simulink model "Test"  (R2019b)
settings: Solver=FixedStepAuto  StartTime=0.0  StopTime=10.0  FixedStep=0.005  RelTol=1e-3
values from neighbouring files (symbols this model uses):
  unbroken = 0    [AplysiaFeeding.m]    (also in AplysiaFeeding_MATLAB.m = 1)
undefined symbols (not defined in the file or in its folder): force_on_object, grasper_friction_state, init_obj, jaw_friction_state, x_g, x_h
(part 1 of 2)
settings Model: Creator=mecha  LastModifiedBy=aslakshm

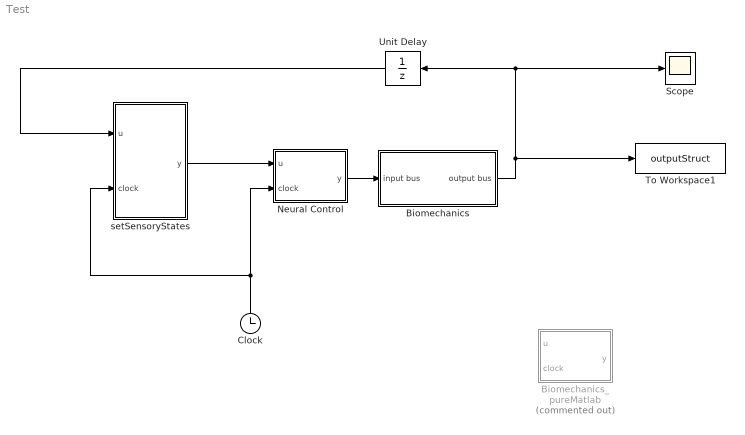
== system Test ==
  Biomechanics : Subsystem
  Biomechanics_pureMatlab : MATLAB Function  Commented=on  TreatAsAtomicUnit=on
  Clock : Clock
  Neural Control : MATLAB Function  TreatAsAtomicUnit=on
  Scope : Scope
  To Workspace1 : ToWorkspace  VariableName=outputStruct  SaveFormat=Timeseries  SampleTime=-1
  Unit Delay : UnitDelay  InitialCondition=init_obj  SampleTime=-1  HasFrameUpgradeWarning=on
  setSensoryStates : MATLAB Function  TreatAsAtomicUnit=on
  wires:
  Clock/1 -> Neural Control/2(clock), setSensoryStates/2(clock)
  Neural Control/1(y) -> Biomechanics/1(input bus)
  Biomechanics/1(output bus) -> To Workspace1/1, Unit Delay/1, Scope/1
  setSensoryStates/1(y) -> Neural Control/1(u)
  Unit Delay/1 -> setSensoryStates/1(u)

== system Test/Biomechanics ==
  input bus : Inport
  Bus Assignment : BusAssignment  AssignedSignals=x_g,x_h,force_on_object,unbroken,jaw_friction_state,grasper_friction_state
  Bus Selector1 : BusSelector  OutputSignals=x_g
  Bus Selector10 : BusSelector  OutputSignals=T_I2
  Bus Selector2 : BusSelector  OutputSignals=x_h
  Bus Selector3 : BusSelector  OutputSignals=fixation_type
  Bus Selector4 : BusSelector  OutputSignals=unbroken
  Bus Selector5 : BusSelector  OutputSignals=sens_mechanical_grasper
  Bus Selector6 : BusSelector  OutputSignals=P_I3_anterior
  Bus Selector7 : BusSelector  OutputSignals=P_I4
  Bus Selector8 : BusSelector  OutputSignals=T_hinge
  Bus Selector9 : BusSelector  OutputSignals=T_I3
  Subsystem : Subsystem
  output bus : Outport
  wires:
  Subsystem/3(Force_On_Object) -> Bus Assignment/4
  Bus Selector1/1 -> Subsystem/1(x_g)  "<x_g>"
  input bus/1 -> Bus Selector10/1, Bus Selector9/1, Bus Selector8/1, Bus Selector7/1, Bus Selector6/1, Bus Selector5/1, Bus Selector4/1, Bus Selector3/1, Bus Selector2/1, Bus Selector1/1, Bus Assignment/1
  Bus Selector2/1 -> Subsystem/2(x_h)  "<x_h>"
  Bus Selector5/1 -> Subsystem/5(sens_mechanical_grasper)  "<sens_mechanical_grasper>"
  Bus Assignment/1 -> output bus/1
  Bus Selector6/1 -> Subsystem/6(P_I3_anterior)  "<P_I3_anterior>"
  Bus Selector7/1 -> Subsystem/7(P_I4)  "<P_I4>"
  Subsystem/2(x_h_out) -> Bus Assignment/3
  Bus Selector3/1 -> Subsystem/3(fixation_type)  "<fixation_type>"
  Subsystem/1(x_g_out) -> Bus Assignment/2
  Bus Selector10/1 -> Subsystem/10(T_I2)  "<T_I2>"
  Bus Selector8/1 -> Subsystem/8(T_hinge)  "<T_hinge>"
  Bus Selector4/1 -> Subsystem/4(unbroken)  "<unbroken>"
  Bus Selector9/1 -> Subsystem/9(T_I3)  "<T_I3>"
  Subsystem/4(unbroken_out) -> Bus Assignment/5
  Subsystem/5(jaw friction state) -> Bus Assignment/6
  Subsystem/6(grasper_friction_state) -> Bus Assignment/7

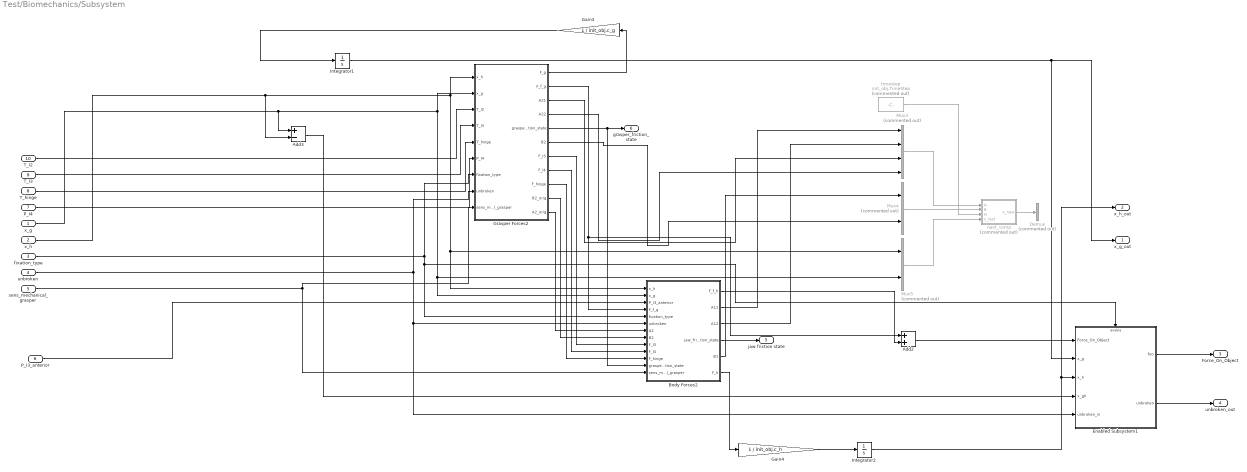
== system Test/Biomechanics/Subsystem ==
  x_g : Inport
  x_h : Inport  Port=2
  fixation_type : Inport  Port=3
  unbroken : Inport  Port=4
  sens_mechanical_grasper : Inport  Port=5
  P_I3_anterior : Inport  Port=6
  P_I4 : Inport  Port=7
  T_hinge : Inport  Port=8
  T_I3 : Inport  Port=9
  T_I2 : Inport  Port=10
  Add2 : Sum
  Add3 : Sum  Inputs=+-
  Body Forces2 : Subsystem
  Demux : Demux  Commented=on  Outputs=2
  Enabled Subsystem1 : Subsystem  TreatAsAtomicUnit=on
  Gain3 : Gain  Gain=1 / init_obj.c_g
  Gain4 : Gain  Gain=1 / init_obj.c_h
  Grasper Forces2 : Subsystem
  Integrator1 : Integrator  InitialCondition=init_obj.x_g_init
  Integrator2 : Integrator  InitialCondition=init_obj.x_h_init
  Mux3 : Mux  Commented=on
  Mux4 : Mux  Commented=on  Inputs=2
  Mux5 : Mux  Commented=on  Inputs=2
  next_comp : MATLAB Function  Commented=on  TreatAsAtomicUnit=on
  timestep : Constant  Commented=on  Value=init_obj.TimeStep
  x_g_out : Outport
  x_h_out : Outport  Port=2
  Force_On_Object : Outport  Port=3
  unbroken_out : Outport  Port=4
  jaw friction state : Outport  Port=5
  grasper_friction_state : Outport  Port=6
  wires:
  P_I4/1 -> Grasper Forces2/6(P_I4)
  Add2/1 -> Enabled Subsystem1/1(Force_On_Object)
  Body Forces2/3(A12) -> Mux3/2
  next_comp/1(x_new) -> Demux/1
  timestep/1 -> next_comp/3(ts)
  Add3/1 -> Enabled Subsystem1/4(x_gh)
  Body Forces2/2(A11) -> Mux3/1
  P_I3_anterior/1 -> Body Forces2/3(P_I3_anterior)
  Mux3/1 -> next_comp/1(A)
  Body Forces2/5(B1) -> Mux4/1
  T_I3/1 -> Grasper Forces2/4(T_I3)
  Grasper Forces2/8(F_I4) -> Body Forces2/10(F_I4)
  unbroken/1 -> Grasper Forces2/8(unbroken), Body Forces2/6(unbroken), Enabled Subsystem1/5(unbroken_in)
  T_hinge/1 -> Grasper Forces2/5(T_hinge)
  fixation_type/1 -> Grasper Forces2/7(fixation_type), Body Forces2/5(fixation_type), Enabled Subsystem1/Enable
  Grasper Forces2/2(F_f_g) -> Body Forces2/4(F_f_g), Add2/1
  Grasper Forces2/7(F_I3) -> Body Forces2/9(F_I3)
  Body Forces2/1(F_f_h) -> Add2/2
  T_I2/1 -> Grasper Forces2/3(T_I2)
  x_g/1 -> Add3/1, Grasper Forces2/2(x_g), Body Forces2/2(x_g), Mux5/2
  Grasper Forces2/10(B2_orig) -> Body Forces2/8(B2)
  sens_mechanical_grasper/1 -> Body Forces2/13(sens_mechanical_grasper), Grasper Forces2/9(sens_mechanical_grasper)
  Grasper Forces2/5(grasper_friction_state) -> Body Forces2/12(grasper_friction_state), grasper_friction_state/1
  Mux4/1 -> next_comp/2(B)
  Grasper Forces2/4(A22) -> Mux3/4
  Grasper Forces2/6(B2) -> Mux4/2
  x_h/1 -> Add3/2, Grasper Forces2/1(x_h), Body Forces2/1(x_h), Mux5/1
  Enabled Subsystem1/1(foo) -> Force_On_Object/1
  Grasper Forces2/3(A21) -> Mux3/3
  Grasper Forces2/11(A2_orig) -> Body Forces2/7(A2)
  Mux5/1 -> next_comp/4(x_last)
  Enabled Subsystem1/2(unbroken) -> unbroken_out/1
  Body Forces2/4(jaw_friction_state) -> jaw friction state/1
  Grasper Forces2/9(F_hinge) -> Body Forces2/11(F_hinge)
  Gain3/1 -> Integrator1/1
  Grasper Forces2/1(F_g) -> Gain3/1
  Integrator1/1 -> Enabled Subsystem1/2(x_g), x_g_out/1
  Body Forces2/6(F_h) -> Gain4/1
  Gain4/1 -> Integrator2/1
  Integrator2/1 -> Enabled Subsystem1/3("x_h "), x_h_out/1

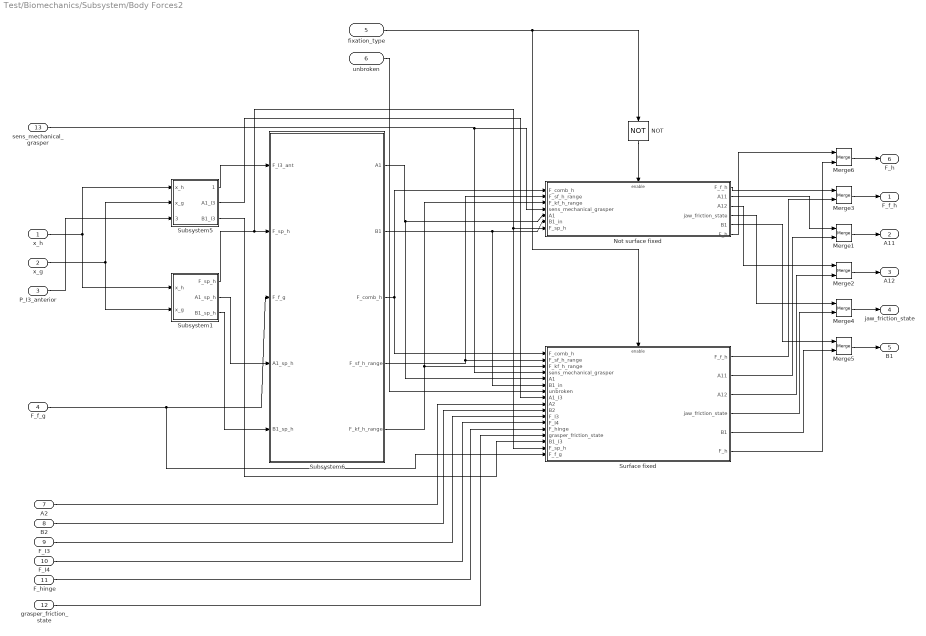
== system Test/Biomechanics/Subsystem/Body Forces2 ==
  x_h : Inport
  x_g : Inport  Port=2
  P_I3_anterior : Inport  Port=3
  F_f_g : Inport  Port=4
  fixation_type : Inport  Port=5
  unbroken : Inport  Port=6
  A2 : Inport  Port=7
  B2 : Inport  Port=8
  F_I3 : Inport  Port=9
  F_I4 : Inport  Port=10
  F_hinge : Inport  Port=11
  grasper_friction_state : Inport  Port=12
  sens_mechanical_grasper : Inport  Port=13
  Merge{1..6} (6 alike) : Merge
  NOT : Logic  Operator=NOT  IconShape=distinctive  AllPortsSameDT=off  OutDataTypeStr=boolean
  Not surface fixed : Subsystem
  Subsystem1 : Subsystem
  Subsystem5 : Subsystem
  Subsystem6 : Subsystem
  Surface fixed : Subsystem
  F_f_h : Outport
  A11 : Outport  Port=2
  A12 : Outport  Port=3
  jaw_friction_state : Outport  Port=4
  B1 : Outport  Port=5
  F_h : Outport  Port=6
  wires:
  Subsystem5/1(F_I3_ant) -> Subsystem6/1(F_I3_ant)
  Subsystem1/1(F_sp_h) -> Surface fixed/16(F_sp_h), Not surface fixed/7(F_sp_h), Subsystem6/2(F_sp_h)
  x_g/1 -> Subsystem1/2(x_g), Subsystem5/2(x_g)
  x_h/1 -> Subsystem1/1(x_h), Subsystem5/1(x_h)
  F_f_g/1 -> Surface fixed/17(F_f_g), Subsystem6/3(F_f_g)
  Subsystem6/4(F_sf_h_range) -> Not surface fixed/2(F_sf_h_range), Surface fixed/2(F_sf_h_range)
  Subsystem6/5(F_kf_h_range) -> Not surface fixed/3(F_kf_h_range), Surface fixed/3(F_kf_h_range)
  Subsystem6/1(A1) -> Surface fixed/5(A1), Not surface fixed/5(A1)
  Subsystem6/3(F_comb_h) -> Surface fixed/1(F_comb_h), Not surface fixed/1(F_comb_h)
  NOT/1 -> Not surface fixed/Enable
  fixation_type/1 -> Surface fixed/Enable, NOT/1
  Merge4/1 -> jaw_friction_state/1
  Merge1/1 -> A11/1
  Merge2/1 -> A12/1
  Merge5/1 -> B1/1
  Merge3/1 -> F_f_h/1
  Surface fixed/5(B1) -> Merge5/2
  Not surface fixed/5(B1) -> Merge5/1
  Surface fixed/4(jaw_friction_state) -> Merge4/2
  Not surface fixed/4(jaw_friction_state) -> Merge4/1
  Surface fixed/3(A12) -> Merge2/2
  Not surface fixed/3(A12) -> Merge2/1
  Surface fixed/2(A11) -> Merge1/2
  Not surface fixed/2(A11) -> Merge1/1
  Surface fixed/1(F_f_h) -> Merge3/2
  Not surface fixed/1(F_f_h) -> Merge3/1
  unbroken/1 -> Surface fixed/7(unbroken)
  Subsystem5/2(A1_I3) -> Surface fixed/8(A1_I3)
  Subsystem5/3(B1_I3) -> Surface fixed/15(B1_I3)
  Subsystem1/2(A1_sp_h) -> Subsystem6/4(A1_sp_h)
  Subsystem1/3(B1_sp_h) -> Subsystem6/5(B1_sp_h)
  A2/1 -> Surface fixed/9(A2)
  B2/1 -> Surface fixed/10(B2)
  grasper_friction_state/1 -> Surface fixed/14(grasper_friction_state)
  Subsystem6/2(B1) -> Surface fixed/6(B1_in), Not surface fixed/6(B1_in)
  P_I3_anterior/1 -> Subsystem5/3(P_I3_anterior)
  F_hinge/1 -> Surface fixed/13(F_hinge)
  F_I3/1 -> Surface fixed/11(F_I3)
  F_I4/1 -> Surface fixed/12(F_I4)
  sens_mechanical_grasper/1 -> Surface fixed/4(sens_mechanical_grasper), Not surface fixed/4(sens_mechanical_grasper)
  Merge6/1 -> F_h/1
  Not surface fixed/6(F_h) -> Merge6/1
  Surface fixed/6(F_h) -> Merge6/2

== system Test/Biomechanics/Subsystem/Enabled Subsystem1 ==
  Force_On_Object : Inport
  x_g : Inport  Port=2
  "x_h " : Inport  Port=3
  x_gh : Inport  Port=4
  unbroken_in : Inport  Port=5
  Enable : EnablePort
  AND : Logic  Inputs=3  IconShape=distinctive  AllPortsSameDT=off  OutDataTypeStr=boolean
  Add : Sum  Inputs=+-
  Constant : Constant  Value=init_obj.seaweed_strength
  Constant1 : Constant  Value=0.3
  Enabled Subsystem : Subsystem  TreatAsAtomicUnit=on
  Enabled Subsystem1 : Subsystem  TreatAsAtomicUnit=on
  GreaterThan : RelationalOperator  Operator=>  OutDataTypeStr=boolean  RndMeth=Simplest
  Less Than : RelationalOperator  Operator=<  OutDataTypeStr=boolean  RndMeth=Simplest
  Less Than1 : RelationalOperator  Operator=>  OutDataTypeStr=boolean  RndMeth=Simplest
  Merge : Merge
  NOT : Logic  Operator=NOT  IconShape=distinctive  AllPortsSameDT=off  OutDataTypeStr=boolean
  NOT1 : Logic  Operator=NOT  IconShape=distinctive  AllPortsSameDT=off  OutDataTypeStr=boolean
  Product : Product
  foo : Outport
  unbroken : Outport  Port=2
  wires:
  Force_On_Object/1 -> Product/1, GreaterThan/1
  Constant/1 -> GreaterThan/2
  x_g/1 -> Add/1
  "x_h "/1 -> Add/2
  x_gh/1 -> Less Than1/2, Less Than/1
  Constant1/1 -> Less Than/2
  Add/1 -> Less Than1/1
  unbroken_in/1 -> Enabled Subsystem1/2(unbroken_in), NOT/1
  Less Than1/1 -> AND/1
  Less Than/1 -> AND/2
  NOT/1 -> AND/3
  AND/1 -> Enabled Subsystem/Enable, NOT1/1
  NOT1/1 -> Enabled Subsystem1/Enable
  GreaterThan/1 -> Enabled Subsystem1/1(force_check)
  Merge/1 -> Product/2, unbroken/1
  Enabled Subsystem1/1(Out1) -> Merge/2
  Enabled Subsystem/1(Out1) -> Merge/1
  Product/1 -> foo/1

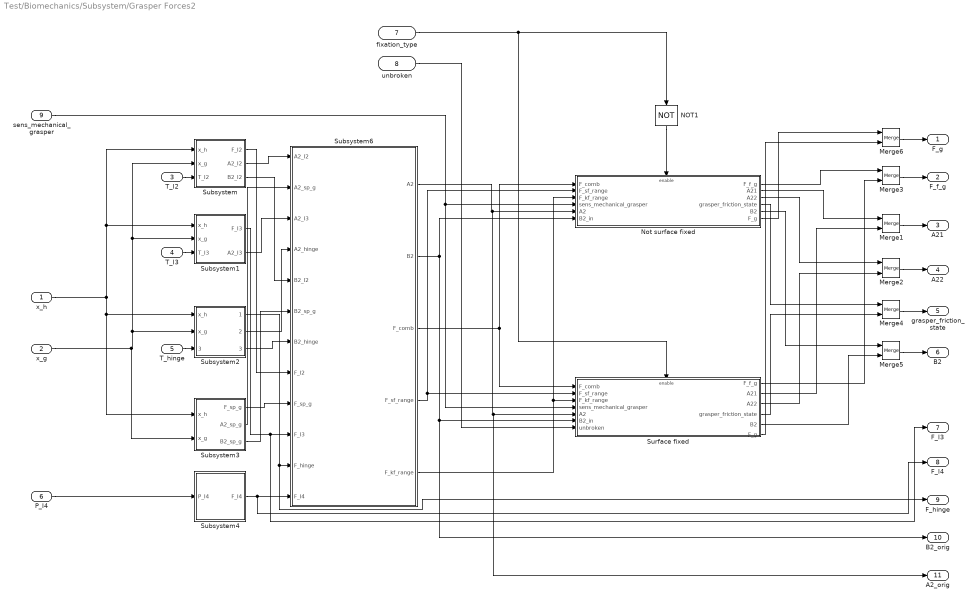
== system Test/Biomechanics/Subsystem/Grasper Forces2 ==
  x_h : Inport
  x_g : Inport  Port=2
  T_I2 : Inport  Port=3
  T_I3 : Inport  Port=4
  T_hinge : Inport  Port=5
  P_I4 : Inport  Port=6
  fixation_type : Inport  Port=7
  unbroken : Inport  Port=8
  sens_mechanical_grasper : Inport  Port=9
  Merge{1..6} (6 alike) : Merge
  NOT1 : Logic  Operator=NOT  IconShape=distinctive  AllPortsSameDT=off  OutDataTypeStr=boolean
  Not surface fixed : Subsystem
  Subsystem : Subsystem
  Subsystem1 : Subsystem
  Subsystem2 : Subsystem
  Subsystem3 : Subsystem
  Subsystem4 : Subsystem
  Subsystem6 : Subsystem
  Surface fixed : Subsystem
  F_g : Outport
  F_f_g : Outport  Port=2
  A21 : Outport  Port=3
  A22 : Outport  Port=4
  grasper_friction_state : Outport  Port=5
  B2 : Outport  Port=6
  F_I3 : Outport  Port=7
  F_I4 : Outport  Port=8
  F_hinge : Outport  Port=9
  B2_orig : Outport  Port=10
  A2_orig : Outport  Port=11
  wires:
  T_hinge/1 -> Subsystem2/3(T_hinge)
  x_h/1 -> Subsystem3/1(x_h), Subsystem2/1(x_h), Subsystem1/1(x_h), Subsystem/1(x_h)
  P_I4/1 -> Subsystem4/1(P_I4)
  x_g/1 -> Subsystem3/2(x_g), Subsystem1/2(x_g), Subsystem/2(x_g), Subsystem2/2(x_g)
  T_I3/1 -> Subsystem1/3(T_I3)
  T_I2/1 -> Subsystem/3(T_I2)
  Subsystem4/1(F_I4) -> F_I4/1, Subsystem6/12(F_I4)
  Subsystem/2(A2_I2) -> Subsystem6/1(A2_I2)
  Subsystem/1(F_I2) -> Subsystem6/8(F_I2)
  Subsystem/3(B2_I2) -> Subsystem6/5(B2_I2)
  Subsystem1/1(F_I3) -> F_I3/1, Subsystem6/10(F_I3)
  Subsystem3/1(F_sp_g) -> Subsystem6/9(F_sp_g)
  Subsystem3/2(A2_sp_g) -> Subsystem6/2(A2_sp_g)
  Subsystem3/3(B2_sp_g) -> Subsystem6/6(B2_sp_g)
  Subsystem2/1(F_hinge) -> F_hinge/1, Subsystem6/11(F_hinge)
  Subsystem2/3(B2_hinge) -> Subsystem6/7(B2_hinge)
  Subsystem2/2(A2_hinge) -> Subsystem6/4(A2_hinge)
  Subsystem1/2(A2_I3) -> Subsystem6/3(A2_I3)
  fixation_type/1 -> Surface fixed/Enable, NOT1/1
  unbroken/1 -> Surface fixed/7(unbroken)
  Subsystem6/1(A2) -> A2_orig/1, Surface fixed/5(A2), Not surface fixed/5(A2)
  Subsystem6/4(F_sf_range) -> Surface fixed/2(F_sf_range), Not surface fixed/2(F_sf_range)
  Subsystem6/5(F_kf_range) -> Not surface fixed/3(F_kf_range), Surface fixed/3(F_kf_range)
  sens_mechanical_grasper/1 -> Surface fixed/4(sens_mechanical_grasper), Not surface fixed/4(sens_mechanical_grasper)
  Merge1/1 -> A21/1
  Merge2/1 -> A22/1
  Merge4/1 -> grasper_friction_state/1
  Not surface fixed/1(F_f_g) -> Merge3/1
  Surface fixed/1(F_f_g) -> Merge3/2
  Not surface fixed/2(A21) -> Merge1/1
  Surface fixed/2(A21) -> Merge1/2
  Not surface fixed/3(A22) -> Merge2/1
  Surface fixed/3(A22) -> Merge2/2
  Not surface fixed/4(grasper_friction_state) -> Merge4/1
  Surface fixed/4(grasper_friction_state) -> Merge4/2
  Not surface fixed/5(B2) -> Merge5/1
  NOT1/1 -> Not surface fixed/Enable
  Subsystem6/2(B2) -> B2_orig/1, Surface fixed/6(B2_in), Not surface fixed/6(B2_in)
  Surface fixed/5(B2) -> Merge5/2
  Merge5/1 -> B2/1
  Subsystem6/3(F_comb) -> Surface fixed/1(F_comb), Not surface fixed/1(F_comb)
  Merge3/1 -> F_f_g/1
  Merge6/1 -> F_g/1
  Surface fixed/6(F_g) -> Merge6/2
  Not surface fixed/6(F_g) -> Merge6/1

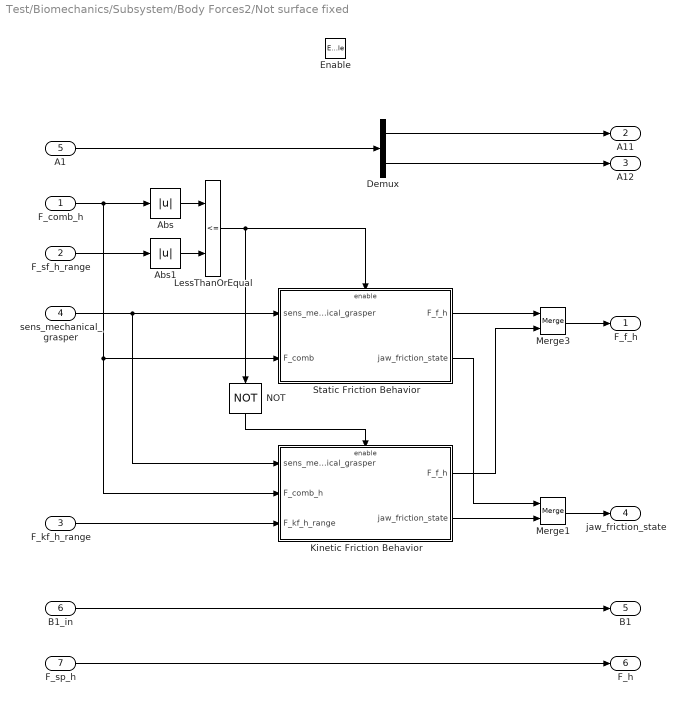
== system Test/Biomechanics/Subsystem/Body Forces2/Not surface fixed ==
  F_comb_h : Inport
  F_sf_h_range : Inport  Port=2
  F_kf_h_range : Inport  Port=3
  sens_mechanical_grasper : Inport  Port=4
  A1 : Inport  Port=5
  B1_in : Inport  Port=6
  F_sp_h : Inport  Port=7
  Enable : EnablePort
  Abs : Abs
  Abs1 : Abs
  Demux : Demux  Outputs=2
  Kinetic Friction Behavior : Subsystem
  LessThanOrEqual : RelationalOperator  Operator=<=  OutDataTypeStr=boolean  RndMeth=Simplest
  Merge1 : Merge
  Merge3 : Merge
  NOT : Logic  Operator=NOT  IconShape=distinctive  AllPortsSameDT=off  OutDataTypeStr=boolean
  Static Friction Behavior : Subsystem
  F_f_h : Outport
  A11 : Outport  Port=2
  A12 : Outport  Port=3
  jaw_friction_state : Outport  Port=4
  B1 : Outport  Port=5
  F_h : Outport  Port=6
  wires:
  A1/1 -> Demux/1
  Demux/2 -> A12/1
  Demux/1 -> A11/1
  F_comb_h/1 -> Kinetic Friction Behavior/2(F_comb_h), Static Friction Behavior/2(F_comb), Abs/1
  F_kf_h_range/1 -> Kinetic Friction Behavior/3(F_kf_h_range)
  F_sf_h_range/1 -> Abs1/1
  Abs/1 -> LessThanOrEqual/1
  Abs1/1 -> LessThanOrEqual/2
  LessThanOrEqual/1 -> NOT/1, Static Friction Behavior/Enable
  NOT/1 -> Kinetic Friction Behavior/Enable
  sens_mechanical_grasper/1 -> Kinetic Friction Behavior/1(sens_mechanical_grasper), Static Friction Behavior/1(sens_mechanical_grasper)
  Static Friction Behavior/1(F_f_h) -> Merge3/1
  Kinetic Friction Behavior/1(F_f_h) -> Merge3/2
  Kinetic Friction Behavior/2(jaw_friction_state) -> Merge1/2
  Static Friction Behavior/2(jaw_friction_state) -> Merge1/1
  Merge3/1 -> F_f_h/1
  Merge1/1 -> jaw_friction_state/1
  B1_in/1 -> B1/1
  F_sp_h/1 -> F_h/1

== system Test/Biomechanics/Subsystem/Body Forces2/Subsystem1 ==
  x_h : Inport
  x_g : Inport  Port=2
  Add2 : Sum
  Constant1 : Constant  Value=init_obj.x_h_ref
  Constant2 : Constant  Value=[-1 0]
  Constant3 : Constant  Value=init_obj.K_sp_h
  Dot Product1 : DotProduct  InputSameDT=on  OutDataTypeStr=Inherit: Inherit via internal rule
  Mux : Mux  Inputs=2
  Product1 : Product
  Product2 : Product
  Product3 : Product
  F_sp_h : Outport
  A1_sp_h : Outport  Port=2
  B1_sp_h : Outport  Port=3
  wires:
  Constant2/1 -> Product1/1, Dot Product1/1
  Dot Product1/1 -> Add2/2
  Mux/1 -> Dot Product1/2
  x_g/1 -> Mux/2
  x_h/1 -> Mux/1
  Product2/1 -> F_sp_h/1
  Add2/1 -> Product2/2
  Constant3/1 -> Product1/2, Product3/2, Product2/1
  Constant1/1 -> Product3/1, Add2/1
  Product1/1 -> A1_sp_h/1
  Product3/1 -> B1_sp_h/1

== system Test/Biomechanics/Subsystem/Body Forces2/Subsystem5 ==
  x_h : Inport
  x_g : Inport  Port=2
  P_I3_anterior : Inport  Port=3
  Add2 : Sum
  Constant1 : Constant
  Constant2 : Constant  Value=[1 -1]
  Constant3 : Constant  Value=init_obj.max_I3ant
  Dot Product : DotProduct  InputSameDT=on  OutDataTypeStr=Inherit: Inherit via internal rule
  Mux : Mux  Inputs=2
  Product1 : Product  Inputs=3
  Product2 : Product  Inputs=3
  Product3 : Product  Inputs=3
  F_I3_ant : Outport
  A1_I3 : Outport  Port=2
  B1_I3 : Outport  Port=3
  wires:
  Dot Product/1 -> Add2/2
  Mux/1 -> Dot Product/2
  x_g/1 -> Mux/2
  x_h/1 -> Mux/1
  Product2/1 -> F_I3_ant/1
  Add2/1 -> Product2/2
  Constant2/1 -> Product1/2, Dot Product/1
  Product1/1 -> A1_I3/1
  P_I3_anterior/1 -> Product3/3, Product1/3, Product2/3
  Constant1/1 -> Product3/2, Add2/1
  Constant3/1 -> Product3/1, Product1/1, Product2/1
  Product3/1 -> B1_I3/1

== system Test/Biomechanics/Subsystem/Body Forces2/Subsystem6 ==
  F_I3_ant : Inport
  F_sp_h : Inport  Port=2
  F_f_g : Inport  Port=3
  A1_sp_h : Inport  Port=4
  B1_sp_h : Inport  Port=5
  Add : Sum
  Gain1 : Gain  Gain=1 / init_obj.c_h
  Gain2 : Gain  Gain=init_obj.mu_s_h
  Gain3 : Gain  Gain=init_obj.mu_k_h
  Gain4 : Gain  Gain=1 / init_obj.c_h
  A1 : Outport
  B1 : Outport  Port=2
  F_comb_h : Outport  Port=3
  F_sf_h_range : Outport  Port=4
  F_kf_h_range : Outport  Port=5
  wires:
  Add/1 -> F_comb_h/1
  F_I3_ant/1 -> Gain2/1, Gain3/1
  Gain2/1 -> F_sf_h_range/1
  Gain3/1 -> F_kf_h_range/1
  F_sp_h/1 -> Add/1
  F_f_g/1 -> Add/2
  Gain4/1 -> A1/1
  A1_sp_h/1 -> Gain4/1
  Gain1/1 -> B1/1
  B1_sp_h/1 -> Gain1/1

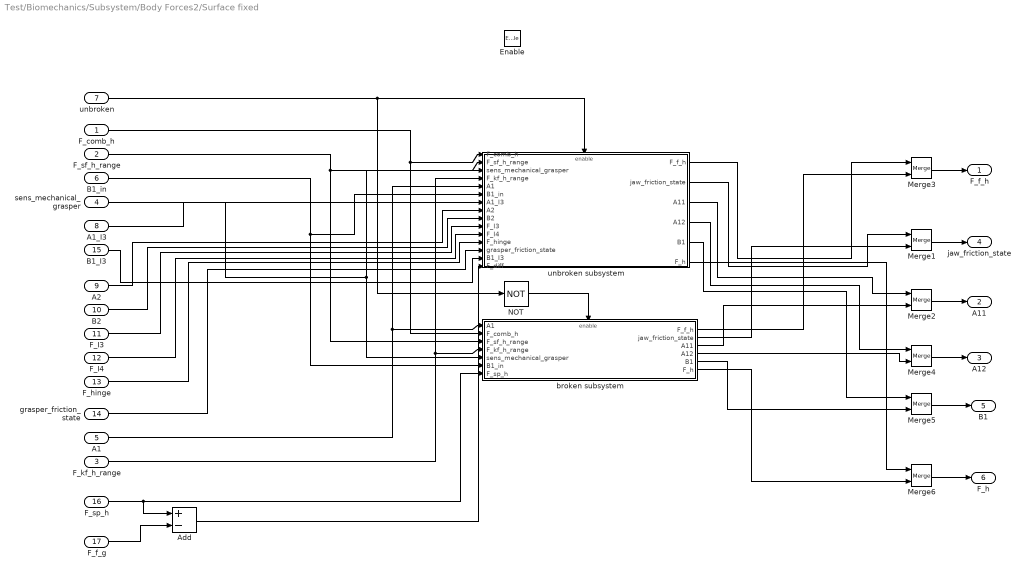
== system Test/Biomechanics/Subsystem/Body Forces2/Surface fixed ==
  F_comb_h : Inport
  F_sf_h_range : Inport  Port=2
  F_kf_h_range : Inport  Port=3
  sens_mechanical_grasper : Inport  Port=4
  A1 : Inport  Port=5
  B1_in : Inport  Port=6
  unbroken : Inport  Port=7
  A1_I3 : Inport  Port=8
  A2 : Inport  Port=9
  B2 : Inport  Port=10
  F_I3 : Inport  Port=11
  F_I4 : Inport  Port=12
  F_hinge : Inport  Port=13
  grasper_friction_state : Inport  Port=14
  B1_I3 : Inport  Port=15
  F_sp_h : Inport  Port=16
  F_f_g : Inport  Port=17
  Enable : EnablePort
  Add : Sum  Inputs=+-
  Merge{1..6} (6 alike) : Merge
  NOT : Logic  Operator=NOT  IconShape=distinctive  AllPortsSameDT=off  OutDataTypeStr=boolean
  broken subsystem : Subsystem
  unbroken subsystem : Subsystem
  F_f_h : Outport
  A11 : Outport  Port=2
  A12 : Outport  Port=3
  jaw_friction_state : Outport  Port=4
  B1 : Outport  Port=5
  F_h : Outport  Port=6
  wires:
  unbroken/1 -> NOT/1, unbroken subsystem/Enable
  NOT/1 -> broken subsystem/Enable
  F_comb_h/1 -> broken subsystem/2(F_comb_h), unbroken subsystem/1(F_comb_h)
  F_sf_h_range/1 -> broken subsystem/3(F_sf_h_range), unbroken subsystem/2(F_sf_h_range)
  A1/1 -> unbroken subsystem/5(A1), broken subsystem/1(A1)
  B1_in/1 -> broken subsystem/6(B1_in), unbroken subsystem/6(B1_in)
  Merge3/1 -> F_f_h/1
  Merge1/1 -> jaw_friction_state/1
  broken subsystem/1(F_f_h) -> Merge3/2
  unbroken subsystem/2(jaw_friction_state) -> Merge1/1
  broken subsystem/2(jaw_friction_state) -> Merge1/2
  Merge2/1 -> A11/1
  Merge4/1 -> A12/1
  unbroken subsystem/3(A11) -> Merge2/1
  broken subsystem/3(A11) -> Merge2/2
  unbroken subsystem/4(A12) -> Merge4/1
  broken subsystem/4(A12) -> Merge4/2
  unbroken subsystem/5(B1) -> Merge5/1
  F_kf_h_range/1 -> unbroken subsystem/4(F_kf_h_range), broken subsystem/4(F_kf_h_range)
  sens_mechanical_grasper/1 -> unbroken subsystem/3(sens_mechanical_grasper), broken subsystem/5(sens_mechanical_grasper)
  Merge5/1 -> B1/1
  broken subsystem/5(B1) -> Merge5/2
  unbroken subsystem/1(F_f_h) -> Merge3/1
  A1_I3/1 -> unbroken subsystem/7(A1_I3)
  A2/1 -> unbroken subsystem/8(A2)
  B2/1 -> unbroken subsystem/9(B2)
  grasper_friction_state/1 -> unbroken subsystem/13(grasper_friction_state)
  B1_I3/1 -> unbroken subsystem/14(B1_I3)
  F_I3/1 -> unbroken subsystem/10(F_I3)
  F_hinge/1 -> unbroken subsystem/12(F_hinge)
  F_I4/1 -> unbroken subsystem/11(F_I4)
  Merge6/1 -> F_h/1
  F_sp_h/1 -> Add/1, broken subsystem/7(F_sp_h)
  broken subsystem/6(F_h) -> Merge6/2
  unbroken subsystem/6(F_h) -> Merge6/1
  F_f_g/1 -> Add/2
  Add/1 -> unbroken subsystem/15(F_diff)

== system Test/Biomechanics/Subsystem/Enabled Subsystem1/Enabled Subsystem ==
  Enable : EnablePort
  Constant : Constant
  Out1 : Outport
  wires:
  Constant/1 -> Out1/1

== system Test/Biomechanics/Subsystem/Enabled Subsystem1/Enabled Subsystem1 ==
  force_check : Inport
  unbroken_in : Inport  Port=2
  Enable : EnablePort
  Enabled Subsystem : Subsystem  TreatAsAtomicUnit=on
  Enabled Subsystem1 : Subsystem  TreatAsAtomicUnit=on
  Merge : Merge
  NOT : Logic  Operator=NOT  IconShape=distinctive  AllPortsSameDT=off  OutDataTypeStr=boolean
  Out1 : Outport
  wires:
  unbroken_in/1 -> Enabled Subsystem1/1(unbroken_in)
  force_check/1 -> NOT/1, Enabled Subsystem/Enable
  NOT/1 -> Enabled Subsystem1/Enable
  Merge/1 -> Out1/1
  Enabled Subsystem1/1(Out1) -> Merge/2
  Enabled Subsystem/1(Out1) -> Merge/1

== system Test/Biomechanics/Subsystem/Grasper Forces2/Not surface fixed ==
  F_comb : Inport
  F_sf_range : Inport  Port=2
  F_kf_range : Inport  Port=3
  sens_mechanical_grasper : Inport  Port=4
  A2 : Inport  Port=5
  B2_in : Inport  Port=6
  Enable : EnablePort
  Abs : Abs
  Abs1 : Abs
  Demux : Demux  Outputs=2
  Kinetic Friction Behavior : Subsystem
  LessThanOrEqual : RelationalOperator  Operator=<=  OutDataTypeStr=boolean  RndMeth=Simplest
  Merge1 : Merge
  Merge3 : Merge
  NOT : Logic  Operator=NOT  IconShape=distinctive  AllPortsSameDT=off  OutDataTypeStr=boolean
  Static Friction Behavior : Subsystem
  F_f_g : Outport
  A21 : Outport  Port=2
  A22 : Outport  Port=3
  grasper_friction_state : Outport  Port=4
  B2 : Outport  Port=5
  F_g : Outport  Port=6
  wires:
  A2/1 -> Demux/1
  Demux/2 -> A22/1
  Demux/1 -> A21/1
  F_comb/1 -> F_g/1, Kinetic Friction Behavior/2(F_comb), Static Friction Behavior/2(F_comb), Abs/1
  F_kf_range/1 -> Kinetic Friction Behavior/3(F_kf_range)
  F_sf_range/1 -> Abs1/1
  Abs/1 -> LessThanOrEqual/1
  Abs1/1 -> LessThanOrEqual/2
  LessThanOrEqual/1 -> NOT/1, Static Friction Behavior/Enable
  NOT/1 -> Kinetic Friction Behavior/Enable
  sens_mechanical_grasper/1 -> Kinetic Friction Behavior/1(sens_mechanical_grasper), Static Friction Behavior/1(sens_mechanical_grasper)
  Static Friction Behavior/1(F_f_g) -> Merge3/1
  Kinetic Friction Behavior/1(F_f_g) -> Merge3/2
  Kinetic Friction Behavior/2(grasper_friction_state) -> Merge1/2
  Static Friction Behavior/2(grasper_friction_state) -> Merge1/1
  Merge3/1 -> F_f_g/1
  Merge1/1 -> grasper_friction_state/1
  B2_in/1 -> B2/1

== system Test/Biomechanics/Subsystem/Grasper Forces2/Subsystem ==
  x_h : Inport
  x_g : Inport  Port=2
  T_I2 : Inport  Port=3
  Add : Sum
  Constant : Constant  Value=init_obj.max_I2
  Constant1 : Constant  Value=[1 -1]
  Constant4 : Constant
  Dot Product : DotProduct  InputSameDT=on  OutDataTypeStr=Inherit: Inherit via internal rule
  Mux : Mux  Inputs=2
  Product : Product  Inputs=3
  Product2 : Product  Inputs=3
  Product3 : Product  Inputs=3
  F_I2 : Outport
  A2_I2 : Outport  Port=2
  B2_I2 : Outport  Port=3
  wires:
  T_I2/1 -> Product3/3, Product2/3, Product/3
  Constant/1 -> Product3/1, Product2/1, Product/1
  Product/1 -> F_I2/1
  x_h/1 -> Mux/1
  x_g/1 -> Mux/2
  Constant1/1 -> Product2/2, Dot Product/1
  Mux/1 -> Dot Product/2
  Constant4/1 -> Product3/2, Add/1
  Add/1 -> Product/2
  Product2/1 -> A2_I2/1
  Product3/1 -> B2_I2/1
  Dot Product/1 -> Add/2

== system Test/Biomechanics/Subsystem/Grasper Forces2/Subsystem1 ==
  x_h : Inport
  x_g : Inport  Port=2
  T_I3 : Inport  Port=3
  Constant1 : Constant  Value=init_obj.max_I3
  Constant2 : Constant  Value=[-1 1]
  Dot Product1 : DotProduct  InputSameDT=on  OutDataTypeStr=Inherit: Inherit via internal rule
  Mux : Mux  Inputs=2
  Product : Product  Inputs=3
  Product2 : Product  Inputs=3
  F_I3 : Outport
  A2_I3 : Outport  Port=2
  wires:
  T_I3/1 -> Product2/3, Product/3
  Constant1/1 -> Product2/1, Product/1
  Product/1 -> F_I3/1
  Mux/1 -> Dot Product1/2
  Dot Product1/1 -> Product/2
  x_g/1 -> Mux/2
  x_h/1 -> Mux/1
  Constant2/1 -> Product2/2, Dot Product1/1
  Product2/1 -> A2_I3/1

== system Test/Biomechanics/Subsystem/Grasper Forces2/Subsystem2 ==
  x_h : Inport
  x_g : Inport  Port=2
  T_hinge : Inport  Port=3
  Add2 : Sum  Inputs=-+
  Constant1 : Constant  Value=[-1 1]
  Constant2 : Constant  Value=init_obj.max_hinge
  Constant3 : Constant  Value=0.5
  Dot Product1 : DotProduct  InputSameDT=on  OutDataTypeStr=Inherit: Inherit via internal rule
  GreaterThan1 : RelationalOperator  Operator=>  OutDataTypeStr=boolean  RndMeth=Simplest
  Mux : Mux  Inputs=2
  Product : Product  Inputs=4
  Product2 : Product  Inputs=4
  Product3 : Product  Inputs=4
  F_hinge : Outport
  A2_hinge : Outport  Port=2
  B2_hinge : Outport  Port=3
  wires:
  T_hinge/1 -> Product/4, Product3/4, Product2/4
  Constant2/1 -> Product/1, Product3/1, Product2/1
  Product/1 -> F_hinge/1
  Constant1/1 -> Product2/2, Dot Product1/1
  x_h/1 -> Mux/1
  x_g/1 -> Mux/2
  Mux/1 -> Dot Product1/2
  Constant3/1 -> Add2/1, Product3/2, GreaterThan1/2
  Dot Product1/1 -> GreaterThan1/1, Add2/2
  Add2/1 -> Product/2
  GreaterThan1/1 -> Product3/3, Product2/3, Product/3
  Product2/1 -> A2_hinge/1
  Product3/1 -> B2_hinge/1

== system Test/Biomechanics/Subsystem/Grasper Forces2/Subsystem3 ==
  x_h : Inport
  x_g : Inport  Port=2
  Add : Sum
  Constant1 : Constant  Value=init_obj.K_sp_g
  Constant2 : Constant  Value=[1 -1]
  Constant4 : Constant  Value=init_obj.x_gh_ref
  Dot Product1 : DotProduct  InputSameDT=on  OutDataTypeStr=Inherit: Inherit via internal rule
  Mux : Mux  Inputs=2
  Product : Product
  Product2 : Product
  Product3 : Product
  F_sp_g : Outport
  A2_sp_g : Outport  Port=2
  B2_sp_g : Outport  Port=3
  wires:
  Product/1 -> F_sp_g/1
  Add/1 -> Product/1
  Constant4/1 -> Product3/1, Add/1
  Constant1/1 -> Product2/2, Product3/2, Product/2
  x_h/1 -> Mux/1
  x_g/1 -> Mux/2
  Constant2/1 -> Product2/1, Dot Product1/1
  Mux/1 -> Dot Product1/2
  Dot Product1/1 -> Add/2
  Product2/1 -> A2_sp_g/1
  Product3/1 -> B2_sp_g/1

== system Test/Biomechanics/Subsystem/Grasper Forces2/Subsystem4 ==
  P_I4 : Inport
  Constant4 : Constant  Value=init_obj.max_I4
  Product : Product
  F_I4 : Outport
  wires:
  P_I4/1 -> Product/2
  Product/1 -> F_I4/1
  Constant4/1 -> Product/1

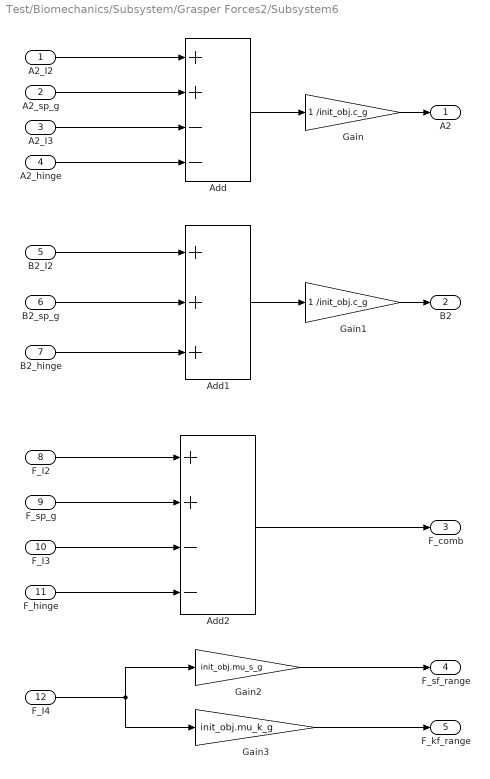
== system Test/Biomechanics/Subsystem/Grasper Forces2/Subsystem6 ==
  A2_I2 : Inport
  A2_sp_g : Inport  Port=2
  A2_I3 : Inport  Port=3
  A2_hinge : Inport  Port=4
  B2_I2 : Inport  Port=5
  B2_sp_g : Inport  Port=6
  B2_hinge : Inport  Port=7
  F_I2 : Inport  Port=8
  F_sp_g : Inport  Port=9
  F_I3 : Inport  Port=10
  F_hinge : Inport  Port=11
  F_I4 : Inport  Port=12
  Add : Sum  Inputs=++--
  Add1 : Sum  Inputs=+++
  Add2 : Sum  Inputs=++--
  Gain : Gain  Gain=1 /init_obj.c_g
  Gain1 : Gain  Gain=1 /init_obj.c_g
  Gain2 : Gain  Gain=init_obj.mu_s_g
  Gain3 : Gain  Gain=init_obj.mu_k_g
  A2 : Outport
  B2 : Outport  Port=2
  F_comb : Outport  Port=3
  F_sf_range : Outport  Port=4
  F_kf_range : Outport  Port=5
  wires:
  A2_sp_g/1 -> Add/2
  A2_hinge/1 -> Add/4
  B2_I2/1 -> Add1/1
  B2_sp_g/1 -> Add1/2
  B2_hinge/1 -> Add1/3
  A2_I3/1 -> Add/3
  A2_I2/1 -> Add/1
  Add/1 -> Gain/1
  Add1/1 -> Gain1/1
  Gain/1 -> A2/1
  Gain1/1 -> B2/1
  F_I2/1 -> Add2/1
  F_sp_g/1 -> Add2/2
  F_I3/1 -> Add2/3
  Add2/1 -> F_comb/1
  F_I4/1 -> Gain3/1, Gain2/1
  Gain2/1 -> F_sf_range/1
  Gain3/1 -> F_kf_range/1
  F_hinge/1 -> Add2/4

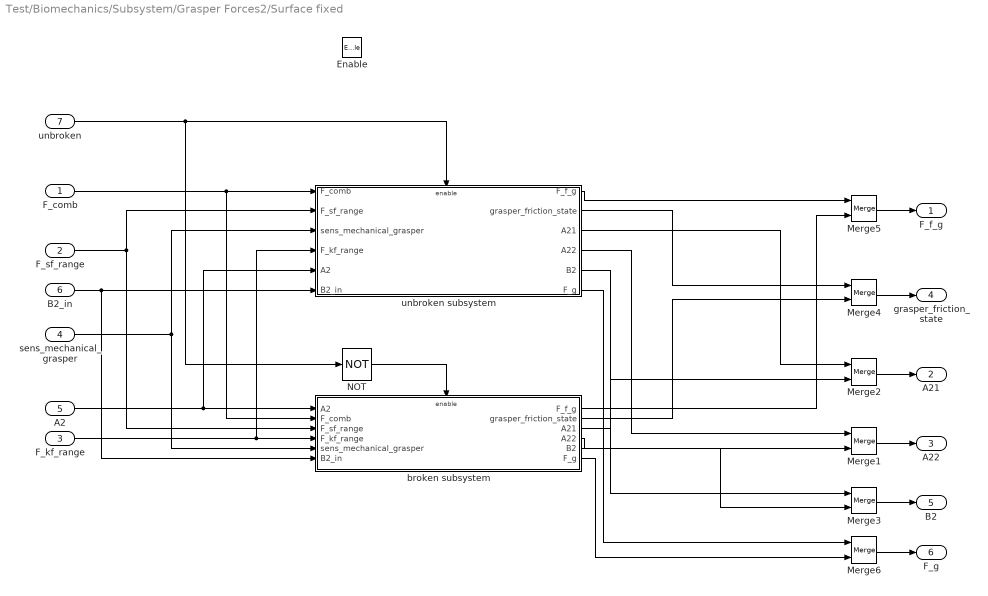
== system Test/Biomechanics/Subsystem/Grasper Forces2/Surface fixed ==
  F_comb : Inport
  F_sf_range : Inport  Port=2
  F_kf_range : Inport  Port=3
  sens_mechanical_grasper : Inport  Port=4
  A2 : Inport  Port=5
  B2_in : Inport  Port=6
  unbroken : Inport  Port=7
  Enable : EnablePort
  Merge{1..6} (6 alike) : Merge
  NOT : Logic  Operator=NOT  IconShape=distinctive  AllPortsSameDT=off  OutDataTypeStr=boolean
  broken subsystem : Subsystem
  unbroken subsystem : Subsystem
  F_f_g : Outport
  A21 : Outport  Port=2
  A22 : Outport  Port=3
  grasper_friction_state : Outport  Port=4
  B2 : Outport  Port=5
  F_g : Outport  Port=6
  wires:
  unbroken/1 -> NOT/1, unbroken subsystem/Enable
  NOT/1 -> broken subsystem/Enable
  F_comb/1 -> broken subsystem/2(F_comb), unbroken subsystem/1(F_comb)
  F_sf_range/1 -> unbroken subsystem/2(F_sf_range), broken subsystem/3(F_sf_range)
  A2/1 -> unbroken subsystem/5(A2), broken subsystem/1(A2)
  B2_in/1 -> broken subsystem/6(B2_in), unbroken subsystem/6(B2_in)
  Merge5/1 -> F_f_g/1
  Merge4/1 -> grasper_friction_state/1
  broken subsystem/1(F_f_g) -> Merge5/2
  unbroken subsystem/2(grasper_friction_state) -> Merge4/1
  broken subsystem/2(grasper_friction_state) -> Merge4/2
  Merge2/1 -> A21/1
  Merge1/1 -> A22/1
  unbroken subsystem/3(A21) -> Merge2/1
  broken subsystem/3(A21) -> Merge2/2
  unbroken subsystem/4(A22) -> Merge1/1
  broken subsystem/4(A22) -> Merge1/2
  unbroken subsystem/5(B2) -> Merge3/1
  F_kf_range/1 -> unbroken subsystem/4(F_kf_range), broken subsystem/4(F_kf_range)
  sens_mechanical_grasper/1 -> broken subsystem/5(sens_mechanical_grasper), unbroken subsystem/3(sens_mechanical_grasper)
  Merge3/1 -> B2/1
  broken subsystem/5(B2) -> Merge3/2
  unbroken subsystem/1(F_f_g) -> Merge5/1
  Merge6/1 -> F_g/1
  broken subsystem/6(F_g) -> Merge6/2
  unbroken subsystem/6(F_g) -> Merge6/1

== system Test/Biomechanics/Subsystem/Body Forces2/Not surface fixed/Kinetic Friction Behavior ==
  sens_mechanical_grasper : Inport
  F_comb_h : Inport  Port=2
  F_kf_h_range : Inport  Port=3
  Enable : EnablePort
  Constant : Constant  Value=0
  Gain1 : Gain  Gain=-1
  Product : Product
  Product1 : Product
  Sign : Signum
  F_f_h : Outport
  jaw_friction_state : Outport  Port=2
  wires:
  Constant/1 -> jaw_friction_state/1
  F_kf_h_range/1 -> Product/2
  Product/1 -> Product1/1
  Product1/1 -> F_f_h/1
  sens_mechanical_grasper/1 -> Product/1
  F_comb_h/1 -> Sign/1
  Sign/1 -> Gain1/1
  Gain1/1 -> Product1/2

== system Test/Biomechanics/Subsystem/Body Forces2/Not surface fixed/Static Friction Behavior ==
  sens_mechanical_grasper : Inport
  F_comb : Inport  Port=2
  Enable : EnablePort
  Constant : Constant
  Gain : Gain  Gain=-1
  Product : Product
  F_f_h : Outport
  jaw_friction_state : Outport  Port=2
  wires:
  Constant/1 -> jaw_friction_state/1
  sens_mechanical_grasper/1 -> Gain/1
  F_comb/1 -> Product/2
  Gain/1 -> Product/1
  Product/1 -> F_f_h/1

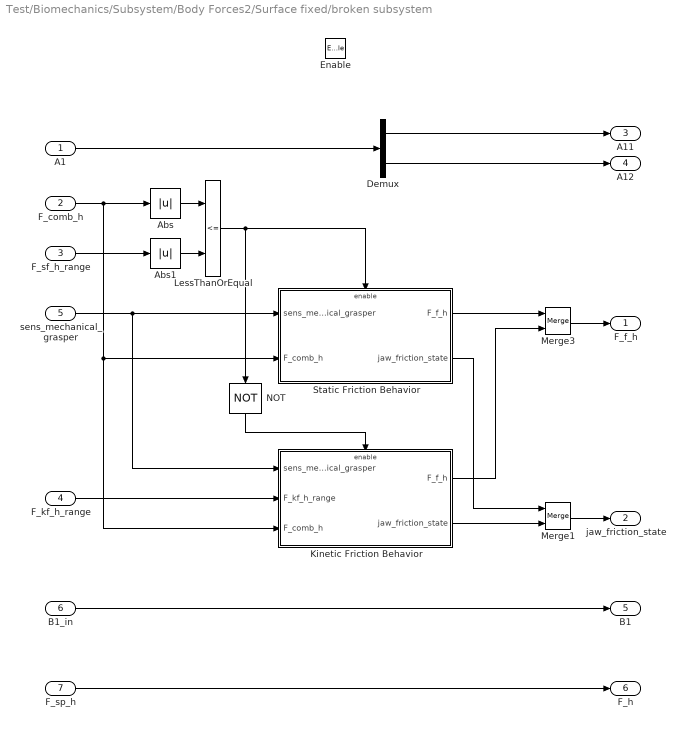
== system Test/Biomechanics/Subsystem/Body Forces2/Surface fixed/broken subsystem ==
  A1 : Inport
  F_comb_h : Inport  Port=2
  F_sf_h_range : Inport  Port=3
  F_kf_h_range : Inport  Port=4
  sens_mechanical_grasper : Inport  Port=5
  B1_in : Inport  Port=6
  F_sp_h : Inport  Port=7
  Enable : EnablePort
  Abs : Abs
  Abs1 : Abs
  Demux : Demux  Outputs=2
  Kinetic Friction Behavior : Subsystem
  LessThanOrEqual : RelationalOperator  Operator=<=  OutDataTypeStr=boolean  RndMeth=Simplest
  Merge1 : Merge
  Merge3 : Merge
  NOT : Logic  Operator=NOT  IconShape=distinctive  AllPortsSameDT=off  OutDataTypeStr=boolean
  Static Friction Behavior : Subsystem
  F_f_h : Outport
  jaw_friction_state : Outport  Port=2
  A11 : Outport  Port=3
  A12 : Outport  Port=4
  B1 : Outport  Port=5
  F_h : Outport  Port=6
  wires:
  A1/1 -> Demux/1
  Demux/2 -> A12/1
  Demux/1 -> A11/1
  F_comb_h/1 -> Kinetic Friction Behavior/3(F_comb_h), Static Friction Behavior/2(F_comb_h), Abs/1
  F_kf_h_range/1 -> Kinetic Friction Behavior/2(F_kf_h_range)
  F_sf_h_range/1 -> Abs1/1
  Abs/1 -> LessThanOrEqual/1
  Abs1/1 -> LessThanOrEqual/2
  LessThanOrEqual/1 -> NOT/1, Static Friction Behavior/Enable
  NOT/1 -> Kinetic Friction Behavior/Enable
  sens_mechanical_grasper/1 -> Kinetic Friction Behavior/1(sens_mechanical_grasper), Static Friction Behavior/1(sens_mechanical_grasper)
  Static Friction Behavior/1(F_f_h) -> Merge3/1
  Kinetic Friction Behavior/1(F_f_h) -> Merge3/2
  Kinetic Friction Behavior/2(jaw_friction_state) -> Merge1/2
  Static Friction Behavior/2(jaw_friction_state) -> Merge1/1
  Merge3/1 -> F_f_h/1
  Merge1/1 -> jaw_friction_state/1
  B1_in/1 -> B1/1
  F_sp_h/1 -> F_h/1

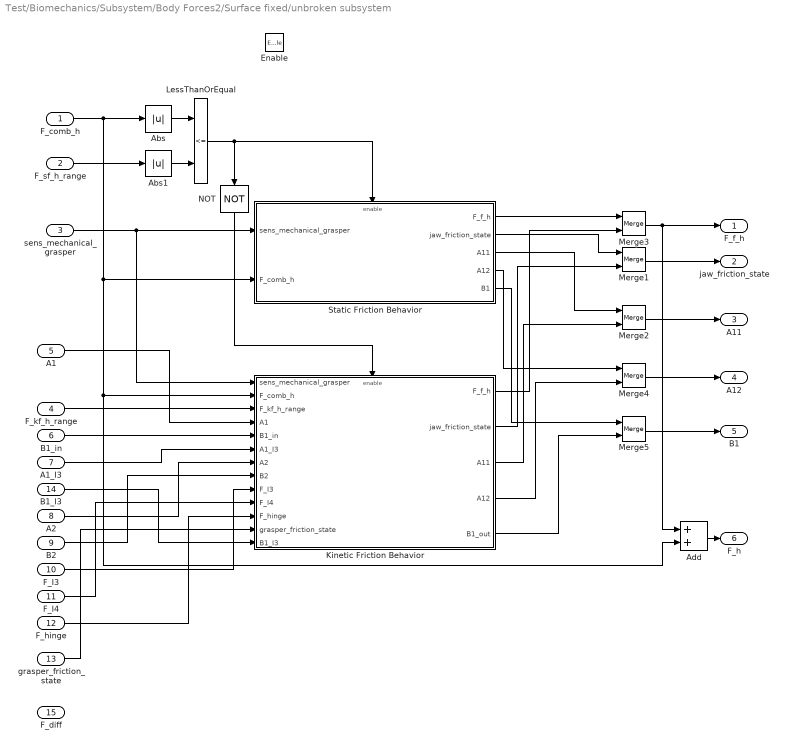
== system Test/Biomechanics/Subsystem/Body Forces2/Surface fixed/unbroken subsystem ==
  F_comb_h : Inport
  F_sf_h_range : Inport  Port=2
  sens_mechanical_grasper : Inport  Port=3
  F_kf_h_range : Inport  Port=4
  A1 : Inport  Port=5
  B1_in : Inport  Port=6
  A1_I3 : Inport  Port=7
  A2 : Inport  Port=8
  B2 : Inport  Port=9
  F_I3 : Inport  Port=10
  F_I4 : Inport  Port=11
  F_hinge : Inport  Port=12
  grasper_friction_state : Inport  Port=13
  B1_I3 : Inport  Port=14
  F_diff : Inport  Port=15
  Enable : EnablePort
  Abs : Abs
  Abs1 : Abs
  Add : Sum
  Kinetic Friction Behavior : Subsystem
  LessThanOrEqual : RelationalOperator  Operator=<=  OutDataTypeStr=boolean  RndMeth=Simplest
  Merge{1..5} (5 alike) : Merge
  NOT : Logic  Operator=NOT  IconShape=distinctive  AllPortsSameDT=off  OutDataTypeStr=boolean
  Static Friction Behavior : Subsystem
  F_f_h : Outport
  jaw_friction_state : Outport  Port=2
  A11 : Outport  Port=3
  A12 : Outport  Port=4
  B1 : Outport  Port=5
  F_h : Outport  Port=6
  wires:
  Abs/1 -> LessThanOrEqual/1
  LessThanOrEqual/1 -> Static Friction Behavior/Enable, NOT/1
  Abs1/1 -> LessThanOrEqual/2
  Merge5/1 -> B1/1
  Merge4/1 -> A12/1
  Merge2/1 -> A11/1
  Merge1/1 -> jaw_friction_state/1
  Static Friction Behavior/1(F_f_h) -> Merge3/1
  Static Friction Behavior/2(jaw_friction_state) -> Merge1/1
  Kinetic Friction Behavior/2(jaw_friction_state) -> Merge1/2
  Static Friction Behavior/3(A11) -> Merge2/1
  Kinetic Friction Behavior/3(A11) -> Merge2/2
  Kinetic Friction Behavior/4(A12) -> Merge4/2
  Static Friction Behavior/5(B1) -> Merge5/1
  Kinetic Friction Behavior/5(B1_out) -> Merge5/2
  A1/1 -> Kinetic Friction Behavior/4(A1)
  B1_in/1 -> Kinetic Friction Behavior/5(B1_in)
  Merge3/1 -> F_f_h/1, Add/1
  F_kf_h_range/1 -> Kinetic Friction Behavior/3(F_kf_h_range)
  sens_mechanical_grasper/1 -> Static Friction Behavior/1(sens_mechanical_grasper), Kinetic Friction Behavior/1(sens_mechanical_grasper)
  Kinetic Friction Behavior/1(F_f_h) -> Merge3/2
  F_comb_h/1 -> Static Friction Behavior/2(F_comb_h), Add/2, Kinetic Friction Behavior/2(F_comb_h), Abs/1
  Static Friction Behavior/4(A12) -> Merge4/1
  A1_I3/1 -> Kinetic Friction Behavior/6(A1_I3)
  A2/1 -> Kinetic Friction Behavior/7(A2)
  B2/1 -> Kinetic Friction Behavior/8(B2)
  grasper_friction_state/1 -> Kinetic Friction Behavior/12(grasper_friction_state)
  B1_I3/1 -> Kinetic Friction Behavior/13(B1_I3)
  F_I4/1 -> Kinetic Friction Behavior/10(F_I4)
  F_I3/1 -> Kinetic Friction Behavior/9(F_I3)
  F_hinge/1 -> Kinetic Friction Behavior/11(F_hinge)
  NOT/1 -> Kinetic Friction Behavior/Enable
  F_sf_h_range/1 -> Abs1/1
  Add/1 -> F_h/1

== system Test/Biomechanics/Subsystem/Enabled Subsystem1/Enabled Subsystem1/Enabled Subsystem ==
  Enable : EnablePort
  Constant : Constant  Value=0
  Out1 : Outport
  wires:
  Constant/1 -> Out1/1

== system Test/Biomechanics/Subsystem/Enabled Subsystem1/Enabled Subsystem1/Enabled Subsystem1 ==
  unbroken_in : Inport
  Enable : EnablePort
  Out1 : Outport
  wires:
  unbroken_in/1 -> Out1/1

== system Test/Biomechanics/Subsystem/Grasper Forces2/Not surface fixed/Kinetic Friction Behavior ==
  sens_mechanical_grasper : Inport
  F_comb : Inport  Port=2
  F_kf_range : Inport  Port=3
  Enable : EnablePort
  Abs : Abs
  Constant : Constant  Value=0
  Divide : Product  Inputs=*/
  Gain : Gain  Gain=-1
  Product : Product
  Product1 : Product
  F_f_g : Outport
  grasper_friction_state : Outport  Port=2
  wires:
  Constant/1 -> grasper_friction_state/1
  F_kf_range/1 -> Product/2
  F_comb/1 -> Abs/1, Gain/1
  Gain/1 -> Divide/1
  Abs/1 -> Divide/2
  Divide/1 -> Product1/2
  Product/1 -> Product1/1
  Product1/1 -> F_f_g/1
  sens_mechanical_grasper/1 -> Product/1

== system Test/Biomechanics/Subsystem/Grasper Forces2/Not surface fixed/Static Friction Behavior ==
  sens_mechanical_grasper : Inport
  F_comb : Inport  Port=2
  Enable : EnablePort
  Constant : Constant
  Gain : Gain  Gain=-1
  Product : Product
  F_f_g : Outport
  grasper_friction_state : Outport  Port=2
  wires:
  Constant/1 -> grasper_friction_state/1
  sens_mechanical_grasper/1 -> Gain/1
  F_comb/1 -> Product/2
  Gain/1 -> Product/1
  Product/1 -> F_f_g/1

== system Test/Biomechanics/Subsystem/Grasper Forces2/Surface fixed/broken subsystem ==
  A2 : Inport
  F_comb : Inport  Port=2
  F_sf_range : Inport  Port=3
  F_kf_range : Inport  Port=4
  sens_mechanical_grasper : Inport  Port=5
  B2_in : Inport  Port=6
  Enable : EnablePort
  Abs : Abs
  Abs1 : Abs
  Demux : Demux  Outputs=2
  Kinetic Friction Behavior : Subsystem
  LessThanOrEqual : RelationalOperator  Operator=<=  OutDataTypeStr=boolean  RndMeth=Simplest
  Merge1 : Merge
  Merge3 : Merge
  NOT : Logic  Operator=NOT  IconShape=distinctive  AllPortsSameDT=off  OutDataTypeStr=boolean
  Static Friction Behavior : Subsystem
  F_f_g : Outport
  grasper_friction_state : Outport  Port=2
  A21 : Outport  Port=3
  A22 : Outport  Port=4
  B2 : Outport  Port=5
  F_g : Outport  Port=6
  wires:
  A2/1 -> Demux/1
  Demux/2 -> A22/1
  Demux/1 -> A21/1
  F_comb/1 -> F_g/1, Kinetic Friction Behavior/2(F_comb), Static Friction Behavior/2(F_comb), Abs/1
  F_kf_range/1 -> Kinetic Friction Behavior/3(F_kf_range)
  F_sf_range/1 -> Abs1/1
  Abs/1 -> LessThanOrEqual/1
  Abs1/1 -> LessThanOrEqual/2
  LessThanOrEqual/1 -> NOT/1, Static Friction Behavior/Enable
  NOT/1 -> Kinetic Friction Behavior/Enable
  sens_mechanical_grasper/1 -> Kinetic Friction Behavior/1(sens_mechanical_grasper), Static Friction Behavior/1(sens_mechanical_grasper)
  Static Friction Behavior/1(F_f_g) -> Merge3/1
  Kinetic Friction Behavior/1(F_f_g) -> Merge3/2
  Kinetic Friction Behavior/2(grasper_friction_state) -> Merge1/2
  Static Friction Behavior/2(grasper_friction_state) -> Merge1/1
  Merge3/1 -> F_f_g/1
  Merge1/1 -> grasper_friction_state/1
  B2_in/1 -> B2/1

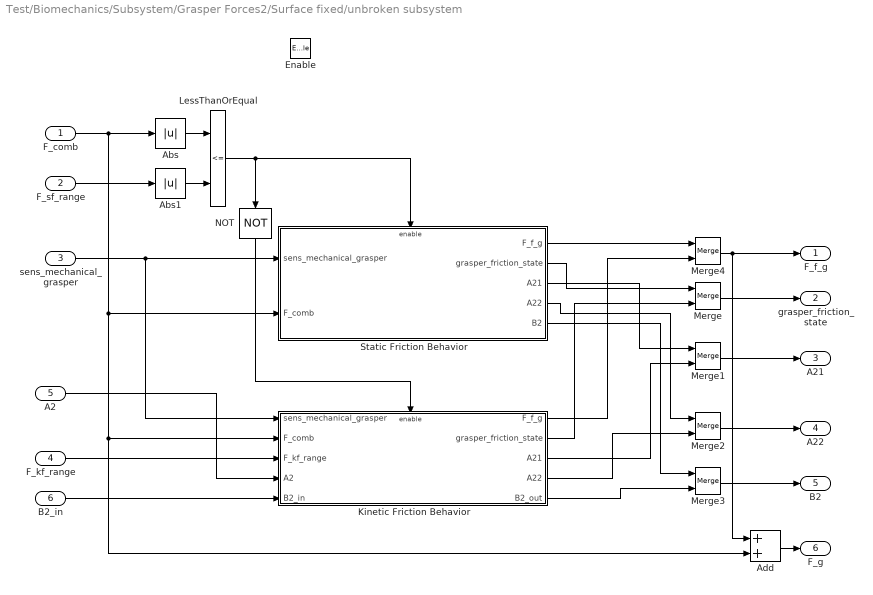
== system Test/Biomechanics/Subsystem/Grasper Forces2/Surface fixed/unbroken subsystem ==
  F_comb : Inport
  F_sf_range : Inport  Port=2
  sens_mechanical_grasper : Inport  Port=3
  F_kf_range : Inport  Port=4
  A2 : Inport  Port=5
  B2_in : Inport  Port=6
  Enable : EnablePort
  Abs : Abs
  Abs1 : Abs
  Add : Sum
  Kinetic Friction Behavior : Subsystem
  LessThanOrEqual : RelationalOperator  Operator=<=  OutDataTypeStr=boolean  RndMeth=Simplest
  Merge{,1..4} (5 alike) : Merge
  NOT : Logic  Operator=NOT  IconShape=distinctive  AllPortsSameDT=off  OutDataTypeStr=boolean
  Static Friction Behavior : Subsystem
  F_f_g : Outport
  grasper_friction_state : Outport  Port=2
  A21 : Outport  Port=3
  A22 : Outport  Port=4
  B2 : Outport  Port=5
  F_g : Outport  Port=6
  wires:
  Abs/1 -> LessThanOrEqual/1
  LessThanOrEqual/1 -> Static Friction Behavior/Enable, NOT/1
  F_sf_range/1 -> Abs1/1
  Abs1/1 -> LessThanOrEqual/2
  NOT/1 -> Kinetic Friction Behavior/Enable
  Merge3/1 -> B2/1
  Merge2/1 -> A22/1
  Merge1/1 -> A21/1
  Merge/1 -> grasper_friction_state/1
  Static Friction Behavior/1(F_f_g) -> Merge4/1
  Static Friction Behavior/2(grasper_friction_state) -> Merge/1
  Kinetic Friction Behavior/2(grasper_friction_state) -> Merge/2
  Static Friction Behavior/3(A21) -> Merge1/1
  Kinetic Friction Behavior/3(A21) -> Merge1/2
  Kinetic Friction Behavior/4(A22) -> Merge2/2
  Static Friction Behavior/5(B2) -> Merge3/1
  Kinetic Friction Behavior/5(B2_out) -> Merge3/2
  A2/1 -> Kinetic Friction Behavior/4(A2)
  B2_in/1 -> Kinetic Friction Behavior/5(B2_in)
  Merge4/1 -> Add/1, F_f_g/1
  F_kf_range/1 -> Kinetic Friction Behavior/3(F_kf_range)
  sens_mechanical_grasper/1 -> Static Friction Behavior/1(sens_mechanical_grasper), Kinetic Friction Behavior/1(sens_mechanical_grasper)
  Kinetic Friction Behavior/1(F_f_g) -> Merge4/2
  F_comb/1 -> Static Friction Behavior/2(F_comb), Add/2, Kinetic Friction Behavior/2(F_comb), Abs/1
  Static Friction Behavior/4(A22) -> Merge2/1
  Add/1 -> F_g/1

== system Test/Biomechanics/Subsystem/Body Forces2/Surface fixed/broken subsystem/Kinetic Friction Behavior ==
  sens_mechanical_grasper : Inport
  F_kf_h_range : Inport  Port=2
  F_comb_h : Inport  Port=3
  Enable : EnablePort
  Constant : Constant  Value=0
  Gain1 : Gain  Gain=-1
  Product : Product
  Product1 : Product
  Sign : Signum
  F_f_h : Outport
  jaw_friction_state : Outport  Port=2
  wires:
  Constant/1 -> jaw_friction_state/1
  F_kf_h_range/1 -> Product/2
  Product/1 -> Product1/1
  Product1/1 -> F_f_h/1
  sens_mechanical_grasper/1 -> Product/1
  F_comb_h/1 -> Sign/1
  Gain1/1 -> Product1/2
  Sign/1 -> Gain1/1

== system Test/Biomechanics/Subsystem/Body Forces2/Surface fixed/broken subsystem/Static Friction Behavior ==
  sens_mechanical_grasper : Inport
  F_comb_h : Inport  Port=2
  Enable : EnablePort
  Constant : Constant
  Gain : Gain  Gain=-1
  Product : Product
  F_f_h : Outport
  jaw_friction_state : Outport  Port=2
  wires:
  Constant/1 -> jaw_friction_state/1
  sens_mechanical_grasper/1 -> Gain/1
  F_comb_h/1 -> Product/2
  Gain/1 -> Product/1
  Product/1 -> F_f_h/1

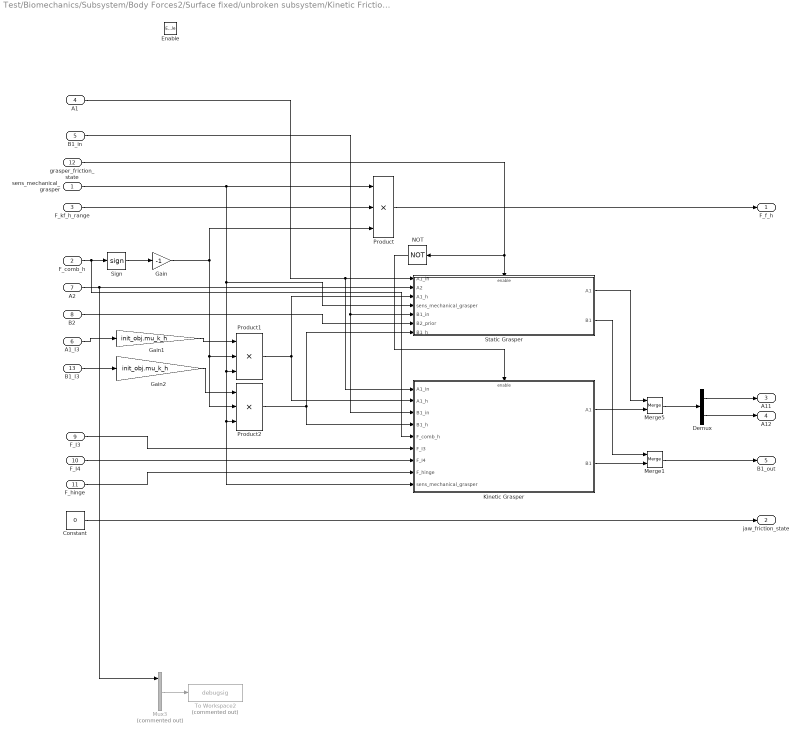
== system Test/Biomechanics/Subsystem/Body Forces2/Surface fixed/unbroken subsystem/Kinetic Friction Behavior ==
  sens_mechanical_grasper : Inport
  F_comb_h : Inport  Port=2
  F_kf_h_range : Inport  Port=3
  A1 : Inport  Port=4
  B1_in : Inport  Port=5
  A1_I3 : Inport  Port=6
  A2 : Inport  Port=7
  B2 : Inport  Port=8
  F_I3 : Inport  Port=9
  F_I4 : Inport  Port=10
  F_hinge : Inport  Port=11
  grasper_friction_state : Inport  Port=12
  B1_I3 : Inport  Port=13
  Enable : EnablePort
  Constant : Constant  Value=0
  Demux : Demux  Outputs=2
  Gain : Gain  Gain=-1
  Gain1 : Gain  Gain=init_obj.mu_k_h
  Gain2 : Gain  Gain=init_obj.mu_k_h
  Kinetic Grasper : Subsystem
  Merge1 : Merge
  Merge5 : Merge
  Mux3 : Mux  Commented=on
  NOT : Logic  Operator=NOT  IconShape=distinctive  AllPortsSameDT=off  OutDataTypeStr=boolean
  Product : Product  Inputs=3
  Product1 : Product  Inputs=3
  Product2 : Product  Inputs=3
  Sign : Signum
  Static Grasper : Subsystem
  To Workspace2 : ToWorkspace  Commented=on  VariableName=debugsig  SaveFormat=Structure With Time  SampleTime=-1
  F_f_h : Outport
  jaw_friction_state : Outport  Port=2
  A11 : Outport  Port=3
  A12 : Outport  Port=4
  B1_out : Outport  Port=5
  wires:
  Constant/1 -> jaw_friction_state/1
  F_comb_h/1 -> Kinetic Grasper/5(F_comb_h), Sign/1
  Product/1 -> F_f_h/1
  F_kf_h_range/1 -> Product/2
  sens_mechanical_grasper/1 -> Static Grasper/4(sens_mechanical_grasper), Kinetic Grasper/9(sens_mechanical_grasper), Product2/3, Product1/3, Product/1
  Sign/1 -> Gain/1
  Gain/1 -> Product2/2, Product1/2, Product/3
  A1_I3/1 -> Gain1/1
  Gain1/1 -> Product1/1
  Merge5/1 -> Demux/1
  Demux/1 -> A11/1
  Demux/2 -> A12/1
  Static Grasper/1(A1) -> Merge5/1
  Kinetic Grasper/1(A1) -> Merge5/2
  Merge1/1 -> B1_out/1
  Kinetic Grasper/2(B1) -> Merge1/2
  Static Grasper/2(B1) -> Merge1/1
  A1/1 -> Kinetic Grasper/1(A1_in), Static Grasper/1(A1_in)
  B1_in/1 -> Static Grasper/5(B1_in), Kinetic Grasper/3(B1_in)
  B2/1 -> Static Grasper/6(B2_prior)
  F_hinge/1 -> Kinetic Grasper/8(F_hinge)
  F_I4/1 -> Kinetic Grasper/7(F_I4)
  F_I3/1 -> Kinetic Grasper/6(F_I3)
  grasper_friction_state/1 -> NOT/1, Static Grasper/Enable
  NOT/1 -> Kinetic Grasper/Enable
  Product1/1 -> Kinetic Grasper/2(A1_h), Static Grasper/3(A1_h)
  B1_I3/1 -> Gain2/1
  Gain2/1 -> Product2/1
  Product2/1 -> Kinetic Grasper/4(B1_h), Static Grasper/7(B1_h)
  Mux3/1 -> To Workspace2/1
  A2/1 -> Mux3/1, Static Grasper/2(A2)

== system Test/Biomechanics/Subsystem/Body Forces2/Surface fixed/unbroken subsystem/Static Friction Behavior ==
  sens_mechanical_grasper : Inport
  F_comb_h : Inport  Port=2
  Enable : EnablePort
  Constant : Constant
  Constant1 : Constant  Value=0
  Gain : Gain  Gain=-1
  Product1 : Product
  F_f_h : Outport
  jaw_friction_state : Outport  Port=2
  A11 : Outport  Port=3
  A12 : Outport  Port=4
  B1 : Outport  Port=5
  wires:
  Constant/1 -> jaw_friction_state/1
  Constant1/1 -> A11/1, A12/1, B1/1
  Product1/1 -> F_f_h/1
  F_comb_h/1 -> Product1/2
  Gain/1 -> Product1/1
  sens_mechanical_grasper/1 -> Gain/1

== system Test/Biomechanics/Subsystem/Grasper Forces2/Surface fixed/broken subsystem/Kinetic Friction Behavior ==
  sens_mechanical_grasper : Inport
  F_comb : Inport  Port=2
  F_kf_range : Inport  Port=3
  Enable : EnablePort
  Abs : Abs
  Constant : Constant  Value=0
  Divide : Product  Inputs=*/
  Gain : Gain  Gain=-1
  Product : Product
  Product1 : Product
  F_f_g : Outport
  grasper_friction_state : Outport  Port=2
  wires:
  Constant/1 -> grasper_friction_state/1
  F_kf_range/1 -> Product/2
  F_comb/1 -> Abs/1, Gain/1
  Gain/1 -> Divide/1
  Abs/1 -> Divide/2
  Divide/1 -> Product1/2
  Product/1 -> Product1/1
  Product1/1 -> F_f_g/1
  sens_mechanical_grasper/1 -> Product/1

== system Test/Biomechanics/Subsystem/Grasper Forces2/Surface fixed/broken subsystem/Static Friction Behavior ==
  sens_mechanical_grasper : Inport
  F_comb : Inport  Port=2
  Enable : EnablePort
  Constant : Constant
  Gain : Gain  Gain=-1
  Product : Product
  F_f_g : Outport
  grasper_friction_state : Outport  Port=2
  wires:
  Constant/1 -> grasper_friction_state/1
  sens_mechanical_grasper/1 -> Gain/1
  F_comb/1 -> Product/2
  Gain/1 -> Product/1
  Product/1 -> F_f_g/1

== system Test/Biomechanics/Subsystem/Grasper Forces2/Surface fixed/unbroken subsystem/Kinetic Friction Behavior ==
  sens_mechanical_grasper : Inport
  F_comb : Inport  Port=2
  F_kf_range : Inport  Port=3
  A2 : Inport  Port=4
  B2_in : Inport  Port=5
  Enable : EnablePort
  Add : Sum
  Constant : Constant  Value=0
  Demux : Demux  Outputs=2
  Gain : Gain  Gain=-1
  Gain1 : Gain  Gain=1 / init_obj.c_g
  Product : Product
  Product1 : Product
  Reshape : Reshape  OutputDimensionality=Customize
  Sign : Signum
  F_f_g : Outport
  grasper_friction_state : Outport  Port=2
  A21 : Outport  Port=3
  A22 : Outport  Port=4
  B2_out : Outport  Port=5
  wires:
  Constant/1 -> grasper_friction_state/1
  F_kf_range/1 -> Product/2
  F_comb/1 -> Sign/1
  sens_mechanical_grasper/1 -> Product/1
  Demux/1 -> A21/1
  A2/1 -> Demux/1
  Demux/2 -> A22/1
  Sign/1 -> Gain/1
  B2_in/1 -> Add/1
  Gain1/1 -> Add/2
  Add/1 -> B2_out/1
  Gain/1 -> Product1/2
  Product/1 -> Product1/1
  Reshape/1 -> Gain1/1, F_f_g/1
  Product1/1 -> Reshape/1

== system Test/Biomechanics/Subsystem/Grasper Forces2/Surface fixed/unbroken subsystem/Static Friction Behavior ==
  sens_mechanical_grasper : Inport
  F_comb : Inport  Port=2
  Enable : EnablePort
  Constant : Constant
  Constant1 : Constant  Value=0
  Gain : Gain  Gain=-1
  Product1 : Product
  F_f_g : Outport
  grasper_friction_state : Outport  Port=2
  A21 : Outport  Port=3
  A22 : Outport  Port=4
  B2 : Outport  Port=5
  wires:
  Constant/1 -> grasper_friction_state/1
  Constant1/1 -> A21/1, A22/1, B2/1
  Product1/1 -> F_f_g/1
  F_comb/1 -> Product1/2
  Gain/1 -> Product1/1
  sens_mechanical_grasper/1 -> Gain/1

== system Test/Biomechanics/Subsystem/Body Forces2/Surface fixed/unbroken subsystem/Kinetic Friction Behavior/Kinetic Grasper ==
  A1_in : Inport
  A1_h : Inport  Port=2
  B1_in : Inport  Port=3
  B1_h : Inport  Port=4
  F_comb_h : Inport  Port=5
  F_I3 : Inport  Port=6
  F_I4 : Inport  Port=7
  F_hinge : Inport  Port=8
  sens_mechanical_grasper : Inport  Port=9
  Enable : EnablePort
  Add : Sum  Inputs=+--  InputSameDT=on
  Add1 : Sum
  Add2 : Sum
  Add3 : Sum
  Gain : Gain  Gain=-1
  Gain1 : Gain  Gain=1 / init_obj.c_h
  Gain2 : Gain  Gain=1 / init_obj.c_h
  Gain3 : Gain  Gain=init_obj.mu_k_g
  Product : Product  Inputs=3
  Sign : Signum
  A1 : Outport
  B1 : Outport  Port=2
  wires:
  A1_h/1 -> Gain2/1
  Gain2/1 -> Add1/2
  A1_in/1 -> Add1/1
  Add1/1 -> A1/1
  F_comb_h/1 -> Add/1
  Add/1 -> Sign/1
  Sign/1 -> Gain/1
  Gain/1 -> Product/2
  Gain3/1 -> Product/3
  sens_mechanical_grasper/1 -> Product/1
  B1_h/1 -> Add2/1
  Add2/1 -> Gain1/1
  Gain1/1 -> Add3/2
  B1_in/1 -> Add3/1
  Add3/1 -> B1/1
  F_I3/1 -> Add/2
  F_hinge/1 -> Add/3
  Product/1 -> Add2/2
  F_I4/1 -> Gain3/1

== system Test/Biomechanics/Subsystem/Body Forces2/Surface fixed/unbroken subsystem/Kinetic Friction Behavior/Static Grasper ==
  A1_in : Inport
  A2 : Inport  Port=2
  A1_h : Inport  Port=3
  sens_mechanical_grasper : Inport  Port=4
  B1_in : Inport  Port=5
  B2_prior : Inport  Port=6
  B1_h : Inport  Port=7
  Enable : EnablePort
  Add{,1..3} (4 alike) : Sum
  Gain : Gain  Gain=init_obj.c_g
  Gain1 : Gain  Gain=-1
  Gain2 : Gain  Gain=1 / init_obj.c_h
  Gain3 : Gain  Gain=init_obj.c_g
  Gain4 : Gain  Gain=1 / init_obj.c_h
  Product : Product
  Product1 : Product
  A1 : Outport
  B1 : Outport  Port=2
  wires:
  A2/1 -> Gain/1
  sens_mechanical_grasper/1 -> Gain1/1
  Gain1/1 -> Product1/1, Product/1
  Gain/1 -> Product/2
  Product/1 -> Add/1
  A1_h/1 -> Add/2
  Add/1 -> Gain2/1
  Gain2/1 -> Add1/2
  A1_in/1 -> Add1/1
  Add1/1 -> A1/1
  B2_prior/1 -> Gain3/1
  Gain3/1 -> Product1/2
  Product1/1 -> Add2/1
  B1_h/1 -> Add2/2
  Add2/1 -> Gain4/1
  Gain4/1 -> Add3/2
  B1_in/1 -> Add3/1
  Add3/1 -> B1/1
